simulink model "simulink_model"  (R2020b)
settings: Solver=VariableStepAuto  StartTime=0.0  StopTime=inf  RelTol=1e-3
libraries: roblocks x2
settings Model: Creator=ramim  LastModifiedBy=nirob

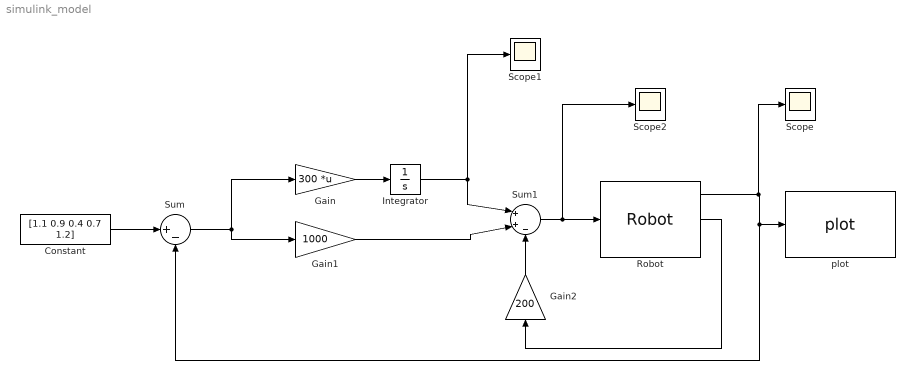
== system simulink_model ==
  Constant : Constant  Value=[1.1 0.9 0.4 0.7 1.2]
  Gain : Gain  Gain=300  Multiplication=Matrix(K*u)
  Gain1 : Gain  Gain=1000
  Gain2 : Gain  Gain=200
  Integrator : Integrator
  Robot : roblocks/Arm/Robot  robot=R  q0=[1 1 1 1 1]*0
  Scope : Scope
  Scope1 : Scope
  Scope2 : Scope
  Sum : Sum  Inputs=|+-
  Sum1 : Sum  Inputs=|++-
  plot : roblocks/Arm/plot  robot=R  fps=50  holdplot=on
  wires:
  Gain/1 -> Integrator/1
  Integrator/1 -> Sum1/1, Scope1/1
  Gain2/1 -> Sum1/3
  Robot/2 -> Gain2/1
  Sum1/1 -> Scope2/1, Robot/1
  Sum/1 -> Gain/1, Gain1/1
  Robot/1 -> Scope/1, plot/1, Sum/2
  Constant/1 -> Sum/1
  Gain1/1 -> Sum1/2
